simulink model "PTBS_ICE_vehicle_DCT"  (R2023b)
settings: Solver=FixedStepAuto  StartTime=0.0  StopTime=1373  FixedStep=0.002  RelTol=1e-3
model workspace (MAT data in the model file):
  Af = 4
  Cd = 0.3
  DownShiftSpeeds = [8.45 25.45 42.45 59.45 76.45 11.25 28.25 45.25 62.25 79.25 14 31 ... (20 elements, 5x4)]
  DrCycles : object (value not decoded)
  I = 5
  Kbr = 500000
  P = 32
  PedalPositions = [10 40 50 90]
  TWAIT = 5
  TimeHWFET = 765
  TimeUDDS = 1372
  TimeUS06 = 596
  UpShiftSpeeds = [11.45 28.45 45.45 62.45 79.45 14.25 31.25 48.25 65.25 82.25 17 34 ... (20 elements, 5x4)]
  axle_b = 10
  axle_k = 5000
  bevAxle_wc = 400
  bevNp = 2
  bevNs = 30
  diffRatio = 3.4
  diffRatio1 = 3.4
  engineSpeedPoints_rpm = [750 1053.57142857 1357.14285714 1660.71428571 1964.28571429 2267.85714286 2571.42857143 2875 3178.57142857 3482.14285714 3785.71428571 4089.28571429 ... (15 elements, 1x15)]
  engineTorqueMap_Nm = [0 15.0034460821 26.4289521305 37.8539339756 49.2854604964 60.7146317399 72.0173711595 77.7345012802 77.7345012802 77.7345012802 77.7345012802 77.7345012802 ... (240 elements, 16x15)]
  engineTorquePoints_Nm = [0 15 26.4285714286 37.8571428571 49.2857142857 60.7142857143 72.1428571429 83.5714285714 95 106.428571429 117.857142857 129.285714286 ... (16 elements, 1x16)]
  motorMaxTorqueNm = [500 500 500 500 500 500 416.666666667 357.142857143 312.5 277.777777778 250 227.272727273 ... (16 elements, 1x16)]
  motorSpeedRadPs = [0 40 80 120 160 200 240 280 320 360 400 440 ... (16 elements, 1x16)]
  vehicleMass = 1500
  wheelRadius = 0.35
libraries: autolibshared x3, autolibsharedcoupling x2, autolibshareddiff x1, slpidlib x1, autolibsharedmappedengines x1, autolibtransdct x1
(part 3 of 5)

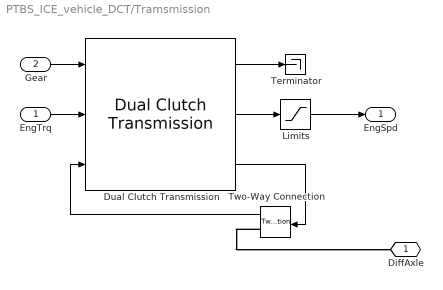
== system PTBS_ICE_vehicle_DCT/Tramsmission ==
  EngTrq : Inport
  Gear : Inport  Port=2
  Dual Clutch Transmission : autolibtransdct/Dual Clutch Transmission  VariantControl=0  cntrlType=Ideal integrated controller  TransEffModelPopup=Gear only  Jin=0.1  bin=0.001  omegain_o=0  G=[-1, 0, 1, 2, 3, 4, 5,6]  Trq_bpts=[25 50 75 100 150 200 250]  omega_bpts=[52.4 78.5 105 131 157 183 209 262 314 419 524]  Temp_bpts=[313 358]  N=[-4.70, 4.70, 4.700, 3.130,2.8, 2.1,1.8, 1.200]  Jout=[0.128 0.01 0.128 0.1 0.062 0.028 0.01 0.01]  bout=[.003 .001 .003 .0025 .002 .001 .001 0.01]  eta=[0.9, 0.9, 0.9, 0.9, 0.9, 0.95, 0.95 0.95]  eta_tbl=reshape([0.57 0.77 0.83 0.86 0.89 0.89 0.89 0.55 0.76 0.83 0.86 0.89 0.89 0.89 0.59 0.78 0.85 0.88 0.9 0.89 0.89 0.61 0.79 0.85 0.88 0.91 0.89 0.89 0.62 0.8 0.86 0.89 0.91 0.89 0.89 0.62 0.8 0.85 0.89 0.91 0.89 0.89 0.63 0.8 0.86 0.89 0.92 0.89 0.89 0.63 0.8 0.86 0.89 0.92 0.89 0.89 0.62 0.81 0.86 0.89 0.92 0.89 0.89 0.6 0.79 0.85 0.88 0.92 0.89 0.89 0.55 0.77 0.84 0.87 0.91 0.89 0.89 0.57 0.77 0.83 0.86 0.89 0.89 0.89 0.55 0.76 0.83 0.86 0.89 0.89 0.89 0.59 0.78 0.85 0.88 0.9 0.89 0.89 0.61 0.79 0.85 0.88 0.91 0.89 0.89 0.62 0.8 0.86 0.89 0.91 0.89 0.89 0.62 0.8 0.85 0.89 0.91 0.89 0.89 0.63 0.8 0.86 0.89 0.92 0.89 0.89 0.63 0.8 0.86 0.89 0.92 0.89 0.89 0.62 0.81 0.86 0.89 0.92 0.89 0.89 0.6 0.79 0.85 0.88 0.92 0.89 0.89 0.55 0.77 0.84 0.87 0.91 0.89 0.89 0.57 0.77 0.83 0.86 0.89 0.89 0.89 0.55 0.76 0.83 0.86 0.89 0.89 0.89 0.59 0.78 0.85 0.88 0.9 0.89 0.89 0.61 0.79 0.85 0.88 0.91 0.89 0.89 0.62 0.8 0.86 0.89 0.91 0.89 0.89 0.62 0.8 0.85 0.89 0.91 0.89 0.89 0.63 0.8 0.86 0.89 0.92 0.89 0.89 0.63 0.8 0.86 0.89 0.92 0.89 0.89 0.62 0.81 0.86 0.89 0.92 0.89 0.89 0.6 0.79 0.85 0.88 0.92 0.89 0.89 0.55 0.77 0.84 0.87 0.91 0.89 0.89 0.76 0.87 0.9 0.91 0.93 0.92 0.92 0.69 0.83 0.88 0.9 0.91 0.92 0.92 0.64 0.81 0.87 0.89 0.91 0.92 0.92 0.63 0.81 0.86 0.89 0.91 0.92 0.92 0.63 0.81 0.86 0.89 0.92 0.92 0.92 0.62 0.8 0.86 0.89 0.92 0.93 0.92 0.62 0.8 0.86 0.89 0.92 0.93 0.92 0.61 0.8 0.86 0.89 0.92 0.93 0.92 0.61 0.8 0.86 0.89 0.92 0.93 0.92 0.57 0.78 0.84 0.88 0.91 0.93 0.92 0.52 0.76 0.83 0.87 0.91 0.93 0.92 0.71 0.84 0.89 0.9 0.92 0.93 0.93 0.62 0.8 0.86 0.89 0.91 0.92 0.93 0.59 0.79 0.85 0.88 0.91 0.92 0.93 0.58 0.79 0.85 0.88 0.91 0.93 0.93 0.57 0.78 0.85 0.88 0.91 0.93 0.94 0.57 0.78 0.85 0.88 0.91 0.93 0.94 0.57 0.78 0.84 0.88 0.91 0.93 0.94 0.55 0.76 0.84 0.87 0.91 0.93 0.94 0.5 0.75 0.83 0.86 0.9 0.92 0.93 0.48 0.74 0.82 0.86 0.9 0.92 0.93 0.41 0.7 0.79 0.83 0.89 0.91 0.92 0.68 0.83 0.88 0.89 0.92 0.93 0.94 0.59 0.78 0.85 0.87 0.9 0.92 0.93 0.54 0.76 0.83 0.87 0.9 0.92 0.93 0.53 0.76 0.83 0.87 0.9 0.92 0.93 0.51 0.75 0.82 0.86 0.9 0.92 0.93 0.5 0.74 0.82 0.86 0.9 0.92 0.93 0.48 0.72 0.81 0.85 0.89 0.91 0.92 0.42 0.7 0.79 0.84 0.88 0.91 0.92 0.31 0.67 0.77 0.82 0.87 0.9 0.91 0.18 0.57 0.7 0.77 0.84 0.87 0.89 0.094 0.47 0.63 0.72 0.81 0.85 0.87 0.68 0.82 0.88 0.89 0.92 0.93 0.93 0.59 0.78 0.84 0.87 0.9 0.92 0.93 0.54 0.76 0.83 0.86 0.9 0.92 0.92 0.53 0.75 0.83 0.86 0.9 0.92 0.93 0.51 0.75 0.82 0.86 0.9 0.92 0.93 0.49 0.74 0.82 0.85 0.89 0.91 0.92 0.47 0.72 0.8 0.85 0.89 0.91 0.92 0.42 0.7 0.79 0.84 0.88 0.9 0.92 0.31 0.67 0.76 0.82 0.87 0.9 0.91 0.18 0.57 0.7 0.77 0.84 0.87 0.89 0.094 0.47 0.63 0.72 0.8 0.85 0.87 0.68 0.82 0.87 0.89 0.91 0.92 0.93 0.59 0.78 0.84 0.87 0.9 0.92 0.93 0.54 0.75 0.83 0.86 0.9 0.91 0.92 0.53 0.75 0.82 0.86 0.9 0.91 0.92 0.51 0.74 0.82 0.86 0.89 0.91 0.92 0.49 0.73 0.81 0.85 0.89 0.91 0.92 0.47 0.72 0.8 0.85 0.89 0.91 0.92 0.42 0.7 0.78 0.83 0.88 0.9 0.91 0.31 0.66 0.76 0.81 0.87 0.89 0.91 0.18 0.57 0.7 0.77 0.83 0.87 0.89 0.093 0.46 0.63 0.72 0.8 0.84 0.87 0.68 0.82 0.87 0.89 0.91 0.92 0.93 0.58 0.78 0.84 0.87 0.9 0.91 0.92 0.54 0.75 0.82 0.86 0.89 0.91 0.92 0.53 0.75 0.82 0.86 0.89 0.91 0.92 0.51 0.74 0.81 0.85 0.89 0.91 0.92 0.49 0.73 0.81 0.85 0.89 0.91 0.92 0.47 0.72 0.8 0.85 0.89 0.91 0.92 0.42 0.69 0.78 0.83 0.88 0.9 0.91 0.31 0.66 0.76 0.81 0.86 0.89 0.9 0.18 0.57 0.69 0.76 0.83 0.87 0.89 0.093 0.46 0.63 0.71 0.8 0.84 0.87 0.67 0.82 0.86 0.88 0.91 0.92 0.92 0.58 0.77 0.83 0.86 0.89 0.91 0.92 0.53 0.75 0.82 0.85 0.89 0.9 0.91 0.52 0.75 0.82 0.85 0.89 0.91 0.92 0.51 0.74 0.81 0.85 0.89 0.91 0.92 0.49 0.73 0.81 0.84 0.88 0.9 0.91 0.47 0.71 0.79 0.84 0.88 0.9 0.91 0.41 0.69 0.78 0.83 0.87 0.89 0.91 0.31 0.66 0.75 0.81 0.86 0.89 0.9 0.18 0.56 0.69 0.76 0.83 0.86 0.88 0.092 0.46 0.63 0.71 0.79 0.84 0.86 0.81 0.88 0.9 0.91 0.92 0.92 0.92 0.75 0.86 0.89 0.91 0.92 0.92 0.92 0.74 0.86 0.89 0.91 0.92 0.92 0.92 0.74 0.86 0.9 0.91 0.93 0.92 0.92 0.74 0.86 0.9 0.91 0.93 0.92 0.92 0.73 0.86 0.89 0.91 0.93 0.92 0.92 ...(+3589 chars))  omegaout_o=0  G_o=0  tauc=.02  ts=.2  tc=.5  R=.25  K_c=5e4  mus=0.3  muk=0.25  ClutchLocked=off  SynchLocked=off  maxAbsSpd=5e3
  Limits : Saturate  UpperLimit=628.3  LowerLimit=52.36
  Terminator : Terminator
  Two-Way Connection : TwoWayConnection
  DiffAxle : PMIOPort  Side=Right
  EngSpd : Outport  Unit=rad/s
  wires:
  Dual Clutch Transmission/3 -> Two-Way Connection/1
  Two-Way Connection/1 -> Dual Clutch Transmission/3
  Gear/1 -> Dual Clutch Transmission/1
  Dual Clutch Transmission/2 -> Limits/1
  Limits/1 -> EngSpd/1
  EngTrq/1 -> Dual Clutch Transmission/2
  Dual Clutch Transmission/1 -> Terminator/1
  connections:
  Two-Way Connection/RConn1 -- DiffAxle/RConn1

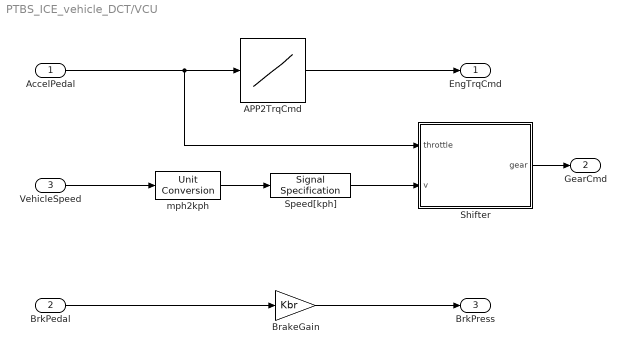
== system PTBS_ICE_vehicle_DCT/VCU ==
  AccelPedal : Inport  Unit=%
  BrkPedal : Inport  Port=2
  VehicleSpeed : Inport  Port=3  Unit=mph
  APP2TrqCmd : Lookup_n-D  NumberOfTableDimensions=1  BreakpointsForDimension1=[ 0 100]  Table=[min(min(engineTorquePoints_Nm)) max(max(engineTorquePoints_Nm))]  ExtrapMethod=Clip  InternalRulePriority=Speed  RndMeth=Simplest
  BrakeGain : Gain  Gain=Kbr
  Shifter : Stateflow chart  TreatAsAtomicUnit=on
  Speed[kph] : SignalSpecification  Unit=km/h
  mph2kph : UnitConversion
  EngTrqCmd : Outport  Unit=N*m
  GearCmd : Outport  Port=2  Unit=1
  BrkPress : Outport  Port=3  Unit=Pa
  wires:
  VehicleSpeed/1 -> mph2kph/1
  BrakeGain/1 -> BrkPress/1
  BrkPedal/1 -> BrakeGain/1
  AccelPedal/1 -> Shifter/1(throttle), APP2TrqCmd/1
  APP2TrqCmd/1 -> EngTrqCmd/1
  Speed[kph]/1 -> Shifter/2(v)
  mph2kph/1 -> Speed[kph]/1
  Shifter/1(gear) -> GearCmd/1

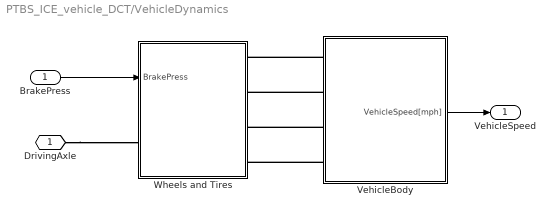
== system PTBS_ICE_vehicle_DCT/VehicleDynamics ==
  BrakePress : Inport
  VehicleBody : Subsystem
  Wheels and Tires : Subsystem
  DrivingAxle : PMIOPort  Side=Left
  VehicleSpeed : Outport
  wires:
  VehicleBody/1(VehicleSpeed[mph]) -> VehicleSpeed/1
  BrakePress/1 -> Wheels and Tires/1(BrakePress)
  connections:
  VehicleBody/LConn4 -- Wheels and Tires/RConn4
  VehicleBody/LConn1 -- Wheels and Tires/RConn1
  VehicleBody/LConn2 -- Wheels and Tires/RConn2
  VehicleBody/LConn3 -- Wheels and Tires/RConn3
  DrivingAxle/RConn1 -- Wheels and Tires/LConn1

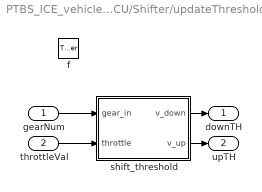
== system PTBS_ICE_vehicle_DCT/VCU/Shifter/updateThresholds ==
  gearNum : Inport  OutDataTypeStr=double  PortDimensions=1
  throttleVal : Inport  Port=2  OutDataTypeStr=double  PortDimensions=1
  f : TriggerPort  TriggerType=function-call  VariantControl=Variant
      settings: CopyFcn=Stateflow.SLINSF.SimulinkMan.removeBlockPreDeleteFcn  PreDeleteFcn=Stateflow.SLINSF.SimulinkMan.unsafePredeleteFcn
  shift_threshold : Subsystem
  downTH : Outport  VectorParamsAs1DForOutWhenUnconnected=off
  upTH : Outport  Port=2  VectorParamsAs1DForOutWhenUnconnected=off
  wires:
  gearNum/1 -> shift_threshold/1(gear_in)
  throttleVal/1 -> shift_threshold/2(throttle)
  shift_threshold/1(v_down) -> downTH/1
  shift_threshold/2(v_up) -> upTH/1

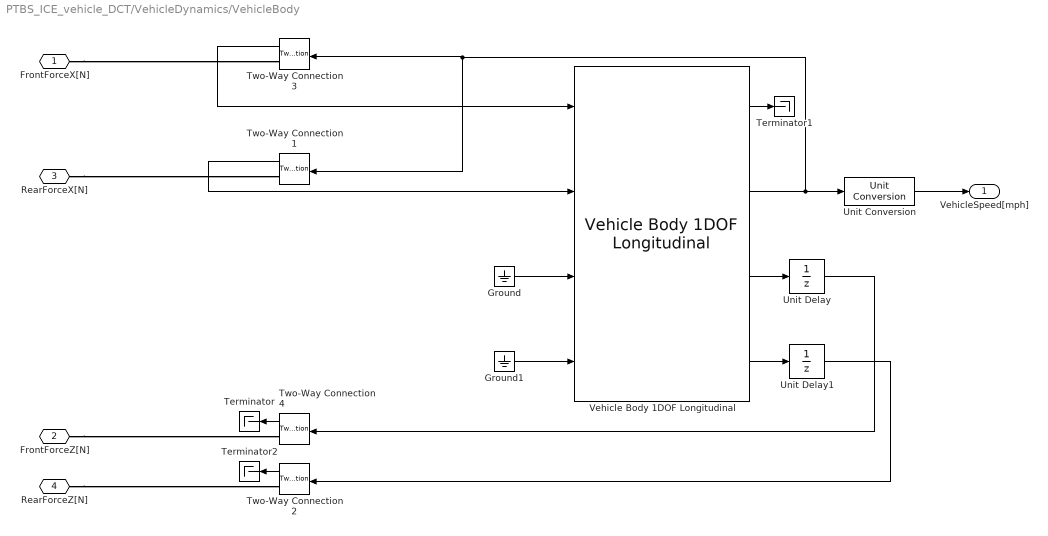
== system PTBS_ICE_vehicle_DCT/VehicleDynamics/VehicleBody ==
  Ground : Ground
  Ground1 : Ground
  Terminator : Terminator
  Terminator1 : Terminator
  Terminator2 : Terminator
  Two-Way Connection{1..4} (4 alike) : TwoWayConnection
  Unit Conversion : UnitConversion
  Unit Delay : UnitDelay  SampleTime=-1  HasFrameUpgradeWarning=on
  Unit Delay1 : UnitDelay  SampleTime=-1  HasFrameUpgradeWarning=on
  Vehicle Body 1DOF Longitudinal : autolibshared/Vehicle Body 1DOF Longitudinal  VariantControl=SL  extFMode=off  extMMode=off  extTamb=off  wind3D=off  aMode=aMode  NF=2  NR=2  m=vehicleMass  a=1.4  b=1.8  h=.35  Cd=.3  Cl=0  Cpm=0  Af=4  x_o=0  xdot_o=0  Pabs=101325  T=273  g=9.81
  FrontForceX[N] : PMIOPort  Side=Left
  FrontForceZ[N] : PMIOPort  Port=2  Side=Left
  RearForceX[N] : PMIOPort  Port=3  Side=Left
  RearForceZ[N] : PMIOPort  Port=4  Side=Left
  VehicleSpeed[mph] : Outport  Unit=mph
  wires:
  Unit Conversion/1 -> VehicleSpeed[mph]/1
  Two-Way Connection3/1 -> Vehicle Body 1DOF Longitudinal/1
  Two-Way Connection4/1 -> Terminator/1
  Two-Way Connection2/1 -> Terminator2/1
  Two-Way Connection1/1 -> Vehicle Body 1DOF Longitudinal/2
  Vehicle Body 1DOF Longitudinal/2 -> Two-Way Connection1/1, Two-Way Connection3/1, Unit Conversion/1
  Vehicle Body 1DOF Longitudinal/1 -> Terminator1/1
  Ground1/1 -> Vehicle Body 1DOF Longitudinal/4
  Ground/1 -> Vehicle Body 1DOF Longitudinal/3
  Vehicle Body 1DOF Longitudinal/3 -> Unit Delay/1
  Vehicle Body 1DOF Longitudinal/4 -> Unit Delay1/1
  Unit Delay/1 -> Two-Way Connection4/1
  Unit Delay1/1 -> Two-Way Connection2/1
  connections:
  FrontForceZ[N]/RConn1 -- Two-Way Connection4/RConn1
  FrontForceX[N]/RConn1 -- Two-Way Connection3/RConn1
  RearForceX[N]/RConn1 -- Two-Way Connection1/RConn1
  RearForceZ[N]/RConn1 -- Two-Way Connection2/RConn1
